simulink model "untitled1"  (R2021b)
settings: Solver=FixedStepAuto  StartTime=0.0  StopTime=Inf  RelTol=1e-3
libraries: robotlib x2
settings Model: Creator=marios  LastModifiedBy=marios
settings OptimizationCC: EnhancedBackFolding=on  PassReuseOutputArgsAs=Individual arguments  ZeroExternalMemoryAtStartup=off  ZeroInternalMemoryAtStartup=off  MaxStackSize=64  OptimizeBlockOrder=speed  DifferentSizesBufferReuse=on  OptimizationCustomize=off  EfficientTunableParamExpr=on
settings DebuggingCC: ParameterTunabilityLossMsg=error
settings HardwareCC: ProdBitPerPointer=32  ProdBitPerSizeT=32  ProdBitPerPtrDiffT=32  ProdLargestAtomicFloat=None  ProdIntDivRoundTo=Undefined  ProdEndianess=Unspecified  ProdWordSize=32  ProdHWDeviceType=Generic->Unspecified (assume 32-bit Generic)
settings SFSimCC: MATLABDynamicMemAlloc=off
settings RTWCC: Description=Embedded Coder  SystemTargetFile=ert.tlc  HardwareBoard=Robot Operating System (ROS)  TLCOptions="-aInlineSetEventsForThisBaseRateFcn=TLC_FALSE -aSuppressMultiTaskScheduler=TLC_FALSE  -aRateBasedStepFcn=0"  TemplateMakefile=ert_default_tmf  Toolchain=Catkin  TargetLang=C++
settings CodeAppCC: ForceParamTrailComments=on  IgnoreCustomStorageClasses=off  OperatorAnnotations=on  SimulinkDataObjDesc=on  SFDataObjDesc=on  InsertBlockDesc=on

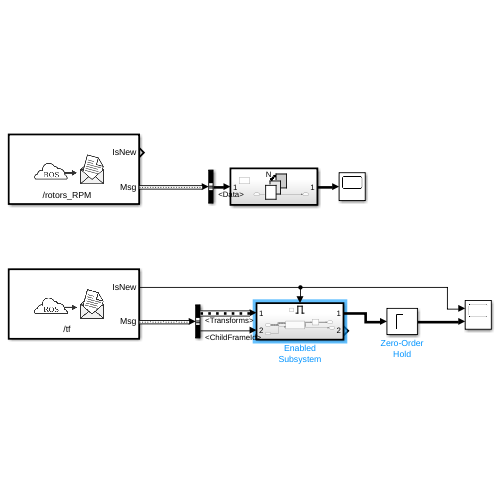
[thumbnail: Simulink's stored preview of the top-level diagram]
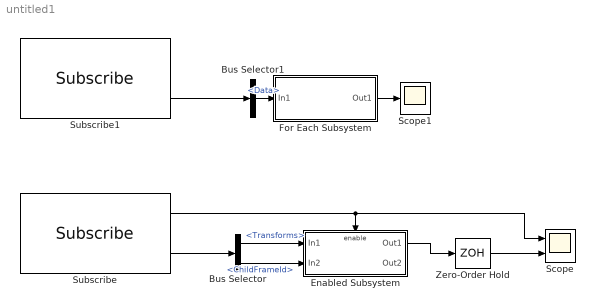
== system untitled1 ==
  Bus Selector : BusSelector  OutputSignals=Transforms,Transforms.ChildFrameId
  Bus Selector1 : BusSelector  OutputSignals=Data
  Enabled Subsystem : Subsystem  TreatAsAtomicUnit=on
  For Each Subsystem : Subsystem  TreatAsAtomicUnit=on
  Scope : Scope  NumInputPorts=2
  Scope1 : Scope
  Subscribe : robotlib/Subscribe  topicSource=Select from ROS network  topic=/tf  messageType=tf2_msgs/TFMessage  SampleTime=-1  legacyBusStruct=off  messageQueueLength=1
  Subscribe1 : robotlib/Subscribe  topicSource=Select from ROS network  topic=/rotors_RPM  messageType=std_msgs/Float32MultiArray  SampleTime=-1  legacyBusStruct=off  messageQueueLength=1
  Zero-Order Hold : ZeroOrderHold  SampleTime=-1
  wires:
  Subscribe/2 -> Bus Selector/1
  Bus Selector/1 -> Enabled Subsystem/1(In1)  "<Transforms>"
  Subscribe/1 -> Scope/1, Enabled Subsystem/Enable
  Enabled Subsystem/1(Out1) -> Zero-Order Hold/1
  Zero-Order Hold/1 -> Scope/2
  Subscribe1/2 -> Bus Selector1/1
  Bus Selector1/1 -> For Each Subsystem/1(In1)  "<Data>"
  For Each Subsystem/1(Out1) -> Scope1/1
  Bus Selector/2 -> Enabled Subsystem/2(In2)  "<ChildFrameId>"

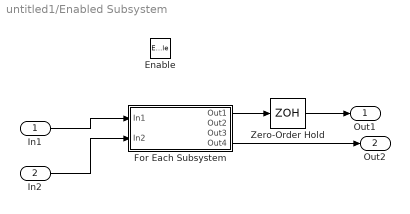
== system untitled1/Enabled Subsystem ==
  In1 : Inport
  In2 : Inport  Port=2
  Enable : EnablePort
  For Each Subsystem : Subsystem  TreatAsAtomicUnit=on
  Zero-Order Hold : ZeroOrderHold  SampleTime=-1
  Out1 : Outport
  Out2 : Outport  Port=2
  wires:
  In1/1 -> For Each Subsystem/1(In1)
  For Each Subsystem/1(Out1) -> Zero-Order Hold/1
  Zero-Order Hold/1 -> Out1/1
  In2/1 -> For Each Subsystem/2(In2)
  For Each Subsystem/4(Out4) -> Out2/1

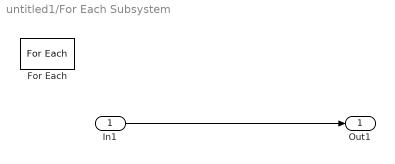
== system untitled1/For Each Subsystem ==
  In1 : Inport  Partition=on  PartitionDimension=1  PartitionWidth=1  PartitionOffset=0
  For Each : ForEach  DisableCoverage=on  SpecifiedNumIters=4
  Out1 : Outport  ConcatenationDimension=1
  wires:
  In1/1 -> Out1/1

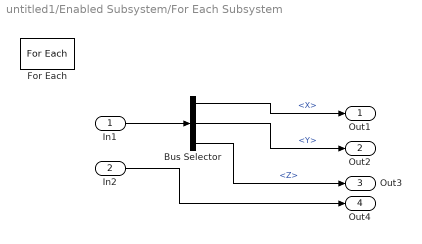
== system untitled1/Enabled Subsystem/For Each Subsystem ==
  In1 : Inport  Partition=on  PartitionDimension=1  PartitionWidth=1  PartitionOffset=0
  In2 : Inport  Port=2
  Bus Selector : BusSelector  OutputSignals=Transform.Translation.X,Transform.Translation.Y,Transform.Translation.Z
  For Each : ForEach  DisableCoverage=on  SpecifiedNumIters=3
  Out1 : Outport  ConcatenationDimension=1
  Out2 : Outport  Port=2  ConcatenationDimension=1
  Out3 : Outport  Port=3  ConcatenationDimension=1
  Out4 : Outport  Port=4  ConcatenationDimension=1
  wires:
  In1/1 -> Bus Selector/1
  Bus Selector/1 -> Out1/1  "<X>"
  Bus Selector/2 -> Out2/1  "<Y>"
  Bus Selector/3 -> Out3/1  "<Z>"
  In2/1 -> Out4/1
